simulink model "BACKUP"  (R2023b)
settings: Solver=VariableStepAuto  StartTime=0.0  StopTime=10.0  RelTol=1e-3
values from neighbouring files (symbols this model uses):
  C_PM = 1.758e-3    (= 0.001758)    [HVDCMMCInterconnectionParam.m]
  Carm = C_PM/Nb_PM    (= 4.88333333333e-05)    [HVDCMMCInterconnectionParam.m]
  Cfilter = 1/(Larm*wc2)    (= 4.78421193241e-05)    [HVDCMMCInterconnectionParam.m]
  Cg = 50e-9    (= 5e-08)    [HVDCMMCInterconnectionParam.m]
  Dd11 = Dd(1:nsw,1:nsw);        if(isempty(Dd11)) Dd11 = zeros(3,3); end    [DSS.m]    (also in DSS_test.m)
  Dd12 = Dd(1:nsw,nsw+1:end);    if(isempty(Dd12)) Dd12 = zeros(3,3); end    [DSS.m]    (also in DSS_test.m)
  Fnom = 50    [HVDCMMCInterconnectionParam.m]
  HRM = 2    [HVDCMMCInterconnectionParam.m]
  Ib_ac = (2/3)*Pnom/Vb_ac    [HVDCMMCInterconnectionParam.m]
  Ki_Ireg = 6    [HVDCMMCInterconnectionParam.m]
  Ki_Preg = 1.0    (= 1)    [HVDCMMCInterconnectionParam.m]
  Ki_Qreg = 1.0    (= 1)    [HVDCMMCInterconnectionParam.m]
  Ki_VDCreg = 100    [HVDCMMCInterconnectionParam.m]
  Kp_Ireg = 0.6    [HVDCMMCInterconnectionParam.m]
  Kp_Preg = 0.5/3    (= 0.166666666667)    [HVDCMMCInterconnectionParam.m]
  Kp_Qreg = 0.5/3    (= 0.166666666667)    [HVDCMMCInterconnectionParam.m]
  Kp_VDCreg = 4    [HVDCMMCInterconnectionParam.m]
  L_cable = 15e-3    (= 0.015)    [HVDCMMCInterconnectionParam.m]
  Larm = Larm_pu*(Zb_ac/(2*pi*Fnom))    [HVDCMMCInterconnectionParam.m]
  Lff = Larm_pu/2    (= 0.075)    [HVDCMMCInterconnectionParam.m]
  Limits_Ireg = [ 2.0  -2.0]    [HVDCMMCInterconnectionParam.m]
  Limits_Preg = [ 1.2, 0.8 ]    [HVDCMMCInterconnectionParam.m]
  Limits_Qreg = [ 0.25, -0.25 ]    [HVDCMMCInterconnectionParam.m]
  Limits_VDCreg = [ 2.0  -2.0]    [HVDCMMCInterconnectionParam.m]
  Lxfo = 0.12    [HVDCMMCInterconnectionParam.m]
  Nb_PM = 36    [HVDCMMCInterconnectionParam.m]
  Pnom = 1000e6    (= 1000000000)    [HVDCMMCInterconnectionParam.m]
  R_cable = 0.5    [HVDCMMCInterconnectionParam.m]
  R_startup = 400    [HVDCMMCInterconnectionParam.m]
  Rarm = Rarm_pu*Zb_ac    [HVDCMMCInterconnectionParam.m]
  Rff = Rarm_pu/2    (= 0.00075)    [HVDCMMCInterconnectionParam.m]
  Rfilter = 1/(Cfilter*w)*30    (= 1996.002)    [HVDCMMCInterconnectionParam.m]
  Rg = 100    [HVDCMMCInterconnectionParam.m]
  Rxfo = 0.003    [HVDCMMCInterconnectionParam.m]
  Ts = Ts_Control    (= 4e-05)    [HVDCMMCInterconnectionParam.m]
  Ts_Control = 40e-6    (= 4e-05)    [HVDCMMCInterconnectionParam.m]
  Ts_Power = 20e-6    (= 2e-05)    [HVDCMMCInterconnectionParam.m]
  Vb_ac = sqrt(2/3)*Vnom_sec    [HVDCMMCInterconnectionParam.m]
  Vc0_PM = 0    [HVDCMMCInterconnectionParam.m]
  Vnom_dc = 640e3    (= 640000)    [HVDCMMCInterconnectionParam.m]
  Vnom_prim = 400e3    (= 400000)    [HVDCMMCInterconnectionParam.m]
  Vnom_sec = 333e3    (= 333000)    [HVDCMMCInterconnectionParam.m]
  w = 2*pi*Fnom    (= 314.159265359)    [HVDCMMCInterconnectionParam.m]
  Zb_ac = Vb_ac/Ib_ac    [HVDCMMCInterconnectionParam.m]
undefined symbols (not defined in the file or in its folder): Ad1, Bd1, Cd1, DiscIntNeverNeededParam, gcbh, HrmOrd, Pcc, sps_AC, sps_ACDC, sps_rtmsupport, SYS, Ts_EMT
libraries: spsSeriesRLCBranchLib x22, simulink x20, spsCurrentMeasurementLib x13, spsControlledVoltageSourceLib x12, DQN_Lib x9, spsdq0toabcLib x3, powerlib_extras x3, spsGroundLib x3, spsBreakerLib x3, spsParallelRLCBranchLib x3, eeGeneralControl x2, dspspect3 x2
(part 2 of 5)

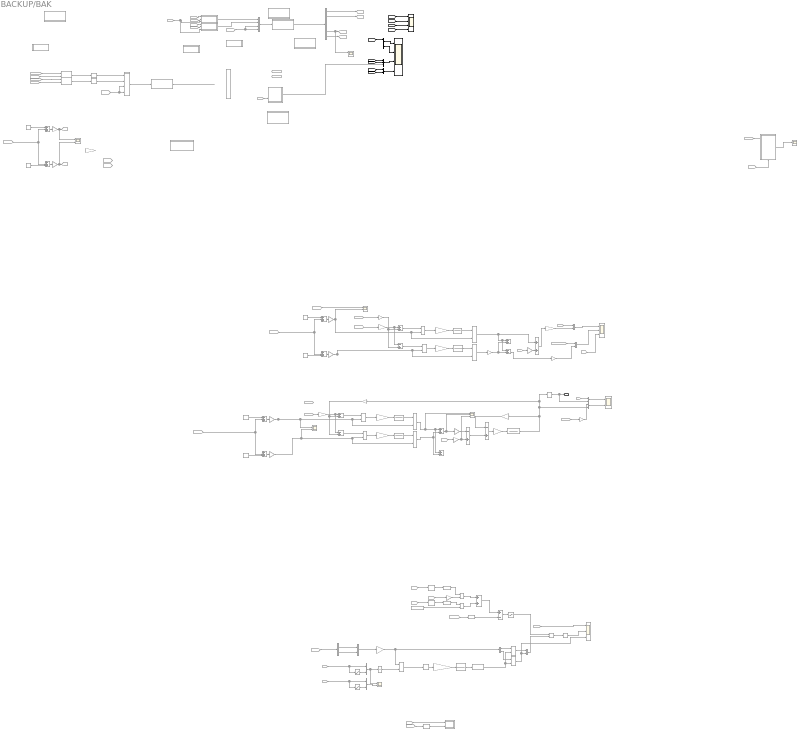
== system BACKUP/BAK ==
  3ph SM1 : Subsystem  Commented=on
  Add{,1,3,7,11} (5 alike) : Sum  Commented=on
  Add2 : Sum  Commented=on  Inputs=-+
  Add4 : Sum  Commented=on  Inputs=+-
  Add6 : Sum  Commented=on  Inputs=-+
  Add9 : Sum  Commented=on  Inputs=-+
  Compare To Constant1 : simulink/Logic and Bit Operations/Compare To Constant  Commented=on  relop=>  const=0.5  OutDataTypeStr=boolean
  Compare To Constant2 : simulink/Logic and Bit Operations/Compare To Constant  Commented=on  relop=<=  const=0.5  OutDataTypeStr=boolean
  Constant{1..4,74..75} (6 alike) : Constant  Commented=on
  Constant5 : Constant  Commented=on  Value=Vb_ac
  DQn->ABC1 : MATLAB Function  Commented=on  TreatAsAtomicUnit=on  SystemSampleTime=Ts_Power  mask{N=HRM}
      mask prompts: N "Harmonic order:"
  Data Type Conversion1 : DataTypeConversion  Commented=on  OutDataTypeStr=double  SaturateOnIntegerOverflow=off  RndMeth=Floor
  Data Type Conversion2 : DataTypeConversion  Commented=on  OutDataTypeStr=double  SaturateOnIntegerOverflow=off  RndMeth=Floor
  Delay : Delay  Commented=on  DelayLength=1  SampleTime=Ts_Power
  Delay1 : Delay  Commented=on  DelayLength=1  SampleTime=Ts_Power
  Delay3 : Subsystem  Commented=on
  Demux : Demux  Commented=on  Outputs=numel(sps_AC.outputs)/3
  Demux11 : Demux  Commented=on  Outputs=2
  Demux9 : Demux  Commented=on  Outputs=2
  Demux_DQNc_Mat : Subsystem  Commented=on  mask{nrOut=numel(sps_AC.outputs)/3}
      mask prompts: nrOut "Number of outputs [{C}]"
      mask init:
      | if(isempty(nrOut))
      |     Simulink.SubSystem.deleteContents(gcb);
      | else
      | 
      |     IndexOptionArray = cell(2,1);
      |     IndexOptionArray(1) = {'Select all'           };
      |     IndexOptionArray(2) = {'Index vector (dialog)'};
      | 
      |     PortHandles = get_param(gcb,'PortHandles');
      | 
      |     lenOut = length(PortHandles.Outport);
      | 
      |     if(nrOut ~= lenOut) % Important to avoid reinitialization of the block!
      | 
      |         Simulink.SubSystem.deleteContents(gcb);
      | 
      |         add_block('built-in/Inport',[gcb,strcat('/In',num2str(1))]);
      |         set_param([gcb,strcat('/In',num2str(1))],'position' , [50,65+1*50,90,85+1*50]);
      | 
      |         for i = 1 : nrOut
      |             add_block('simulink/Signal Routing/Selector',[gcb,strcat('/Sel',num2str(i))],...
      |                 'IndexOptionArray',IndexOptionArray,...
      |                 'NumberOfDimensions','2',...
      |                 'IndexOptions','Index vector (dialog),Select all',...
      |                 'Indices',strcat(num2str((i-1)*3+1),':',num2str((i-1)*3+3),', 1') ...
      |                 );
      |             set_param([gcb,strcat('/Sel',num2str(i))],'position' , [450,65+i*50,490,85+i*50])
      | 
      | 
      |             add_block('built-in/Outport',[gcb,strcat('/Out',num2str(i))]);
      |             set_param([gcb,strcat('/Out',num2str(i))],'position' , [750,65+i*50,790,85+i*50]);
      | 
      |             add_line(gcb,strcat('In',num2str(1),'/1'),  strcat('Sel',num2str(i),'/1'),'autorouting','on');
      |             add_line(gcb,strcat('Sel',num2str(i),'/1'), strcat('Out',num2str(i),'/1'),'autorouting','on');
      |         end
      | 
      |     end
      | 
      | end
      mask Display: disp(['{\color{red}\bf\fontsize{12}} [\{X_C\}]',newline,' DE-',newline,' MUX'], 'texmode','on');
  Discrete State-Space : Subsystem  Commented=on  mask{A=sps_AC.A, B=sps_AC.B, C=sps_AC.C, D=sps_AC.D, InitVec=sps_AC.x0, dt=Ts_Power}
      mask prompts: InitVec "Initial condition:"; dt "Time step (s):"
      mask init:
      | I = eye(size(A,1));
      | INVR = I/(I-A*dt/2);
      | Ad1 = INVR*(I+A*dt/2);
      | Bd1 = INVR*B*dt/2;
      | Cd1 = C*Ad1;
      | Dd11 = C*INVR*B*dt/2+D;
      | Dd12 = C*INVR*B*dt/2;
      settings: LibrarySourceBlock=|
      | spsSynchronousMachineModel/Discrete robust/State Space Model/Discretize
      | BE or Tustin
      mask Display: disp(['{\color{red}\bf\fontsize{12}x(t) = Ad*x(t-dt)+Bd*u(t)}',newline,'{\color{gray}\bf\fontsize{12}y(t) = Cd*x(t-dt)+Dd*u(t)}'], 'texmode','on');
  Discrete State-Space1 : Subsystem  Commented=on  mask{A=sps_AC.A, B=sps_AC.B, C=sps_AC.C, D=sps_AC.D, InitVec=sps_AC.x0, dt=Ts_Power}
      mask prompts: InitVec "Initial condition:"; dt "Time step (s):"
      mask init:
      | % I = eye(size(A,1));
      | % INVR = I/(I-A*dt/2);
      | % Ad1 = INVR*(I+A*dt/2);
      | % Bd1 = INVR*B*dt/2;
      | % Cd1 = C*Ad1;
      | % Cd = INVR*C*dt;
      | % Dd11 = C*INVR*B*dt/2+D;
      | % Dd12 = C*INVR*B*dt/2;
      settings: LibrarySourceBlock=|
      | spsSynchronousMachineModel/Discrete robust/State Space Model/Discretize
      | BE or Tustin
      mask Display: disp(['{\color{red}\bf\fontsize{12}x(t) = Ad*x(t-dt)+Bd*u(t)}',newline,'{\color{gray}\bf\fontsize{12}y(t) = Cd*x(t-dt)+Dd*u(t)}'], 'texmode','on');
  Discrete State-Space2 : Subsystem  Commented=on  mask{A=sps_AC.A, B=sps_AC.B, C=sps_AC.C, D=sps_AC.D, InitVec=[], dt=Ts, N=HRM, Ws=w}
      mask prompts: InitVec "Initial condition:"; dt "Time step (s):"; N "Order number:"; Ws "Angular frequency (rad/s);"
      mask init:
      | %Discretization of Continuous-Time Systems in the State Space with Numerical Integration Methods
      | 
      | method = 1;
      | 
      | % if(method)
      | % 
      | %     I = eye(size(A,1));
      | %     INVR = I/(I-A*dt/2);
      | %     Ad1 = INVR*(I+A*dt/2);
      | %     Bd1 = INVR*B*dt/2;
      | %     Cd1 = C*Ad1;
      | %     Dd1 = C*INVR*B*dt/2+D;
      | %     Dd12 = C*INVR*B*dt/2;
      | % 
      | % else
      | %     I = eye(size(A,1));
      | %     INVR = I/(I-A*dt/2);
      | %     Ad1 = INVR*(I+A*dt/2);
      | %     Bd1 = INVR*B;
      | %     Cd1 = C*INVR*dt;
      | %     Dd1 = Cd1*B/2;
      | % end
      | 
      |     if(method)
      | 
      |         I = eye(size(A,1));
      |         INVR = I/(I-A*dt/2);
      |         Ad1 = INVR*(I+A*dt/2);
      |         Bd1 = INVR*B;
      |         Cd1 = C*INVR*dt;
      |         Dd1 = Cd1*B/2;
      |     else
      |         Ad1 = A;
      |         Bd1 = B;
      |         Cd1 = C;
      |         Dd1 = D;
      |     end
      | 
      | %Calculating the PNZ matrices
      | 
      |     a = -0.5+0.866i;
      |     a2 = -0.5-0.866i;
      |     Sas = [1,a,a2;1,a2,a;1,1,1]/3;
      | 
      |     arows = size(Ad1,1)/3; %signal size
      |     acols = size(Ad1,2)/3; %signal size
      | 
      |     brows = size(Bd1,1)/3; %signal size
      |     bcols = size(Bd1,2)/3; %signal size
      | 
      |     crows = size(Cd1,1)/3; %signal size
      |     ccols = size(Cd1,2)/3; %signal size
      | 
      |     d1rows = size(Dd1,1)/3; %signal size
      |     d1cols = size(Dd1,2)/3; %signal size
      | 
      |     %%%%%%%%%%%%%%%%%%%%%%% Check for inconsistencies  %%%%%%%%%%%%%%%%%%%%%%%
      | 
      |     szMatA = size(A,1);
      |     iL = eye(szMatA);
      |     szMatiL = size(iL,1);
      | 
      |     if(szMatiL ~= szMatA || size(A,1) ~= size(A,2) || size(iL,1) ~= size(iL,2))
      |         error('[Int_DQN_Mat/swFeedback] check matrix A size!');
      |     end
      | 
      |     if(arows ~= brows || acols ~= ccols || crows ~= d1rows || bcols ~= d1cols)
      |         error('[Int_DQN_Mat/Initialize] the sizes of the state-space matrices!');
      |     end
      | 
      |     %%%%%%%%%%%%%%%%%%%%%%%%%%%%%%%%%%%%%%%%%%%%%%%%%%%%%%%%%%%%%%%
      | 
      | 
      |     %%%%%%%%%%%%%%%%%%%%%%% A --> Bpnz %%%%%%%%%%%%%%%%%%%%%%%
      |     Adc = complex(zeros(3*arows,3*acols));
      | 
      |     for i = 1 : arows
      |         for j = 1 : acols
      |             Adc((1:3) + (i-1)*3,(1:3) + (j-1)*3) = Sas*Ad1((1:3) + (i-1)*3,(1:3) + (j-1)*3)/Sas;
      |             %Adc((1:3) + (i-1)*3,(1:3) + (j-1)*3) = diag(diag(real(Adc((1:3) + (i-1)*3,(1:3) + (j-1)*3))));
      |             %Adc((1:3) + (i-1)*3,(1:3) + (j-1)*3) = diag(diag((Adc((1:3) + (i-1)*3,(1:3) + (j-1)*3))));
      | 
      |         end
      |     end
      |     %%%%%%%%%%%%%%%%%%%%%%%%%%%%%%%%%%%%%%%%%%%%%%%%%%%%%%%%%%%%%%%
      | 
      |     %%%%%%%%%%%%%%%%%%%%%%% B --> Bpnz %%%%%%%%%%%%%%%%%%%%%%%
      | 
      |     Bdc = complex(zeros(3*brows,3*bcols));
      | 
      |     for i = 1 : brows
      |         for j = 1 : bcols
      |             Bdc((1:3) + (i-1)*3,(1:3) + (j-1)*3) = Sas*Bd1((1:3) + (i-1)*3,(1:3) + (j-1)*3)/Sas;
      |             %Bdc((1:3) + (i-1)*3,(1:3) + (j-1)*3) = diag(diag(real(Bdc((1:3) + (i-1)*3,(1:3) + (j-1)*3))));
      |             %Bdc((1:3) + (i-1)*3,(1:3) + (j-1)*3) = diag(diag((Bdc((1:3) + (i-1)*3,(1:3) + (j-1)*3))));
      | 
      |         end
      |     end
      |     %%%%%%%%%%%%%%%%%%%%%%%%%%%%%%%%%%%%%%%%%%%%%%%%%%%%%%%%%%%%%%%
      | 
      |     %%%%%%%%%%%%%%%%%%%%%%% C --> Cpnz %%%%%%%%%%%%%%%%%%%%%%%
      | 
      |     Cdc = complex(zeros(3*crows,3*ccols));
      | 
      |     for i = 1 : crows
      |         for j = 1 : ccols
      |             Cdc((1:3) + (i-1)*3,(1:3) + (j-1)*3) = Sas*Cd1((1:3) + (i-1)*3,(1:3) + (j-1)*3)/Sas;
      |             %Cdc((1:3) + (i-1)*3,(1:3) + (j-1)*3) = diag(diag(real(Cdc((1:3) + (i-1)*3,(1:3) + (j-1)*3))));
      |             %Cdc((1:3) + (i-1)*3,(1:3) + (j-1)*3) = diag(diag((Cdc((1:3) + (i-1)*3,(1:3) + (j-1)*3))));
      |         end
      |     end
      |     %%%%%%%%%%%%%%%%%%%%%%%%%%%%%%%%%%%%%%%%%%%%%%%%%%%%%%%%%%%%%%%
      | 
      |     
      |     %%%%%%%%%%%%%%%%%%%%%%% D1 --> Cpnz %%%%%%%%%%%%%%%%%%%%%%%
      | 
      |     Ddc = complex(zeros(3*d1rows,3*d1cols));
      | 
      |     for i = 1 : d1rows
      |         for j = 1 : d1cols
      |             Ddc((1:3) + (i-1)*3,(1:3) + (j-1)*3) = Sas*Dd1((1:3) + (i-1)*3,(1:3) + (j-1)*3)/Sas;
      |             %Ddc1((1:3) + (i-1)*3,(1:3) + (j-1)*3) = diag(diag(real(Ddc1((1:3) + (i-1)*3,(1:3) + (j-1)*3))));
      |             %Ddc((1:3) + (i-1)*3,(1:3) + (j-1)*3) = diag(diag((Ddc((1:3) + (i-1)*3,(1:3) + (j-1)*3))));
      |         end
      |     end
      |     %%%%%%%%%%%%%%%%%%%%%%%%%%%%%%%%%%%%%%%%%%%%%%%%%%%%%%%%%%%%%%%
      | 
      |     Adc(abs(Adc)<2*eps) = 0;
      |     Bdc(abs(Bdc)<2*eps) = 0;
      |     Cdc(abs(Cdc)<2*eps) = 0;
      |     Ddc(abs(Ddc)<2*eps) = 0;
      | 
      |     % I = eye(size(Adc,1));
      |     % INVR = I/(I-Adc*dt/2);
      |     % Adc = INVR*(I+Adc*dt/2);
      |     % Bdc = INVR*Bdc;
      |     % Cdc = Cdc*INVR*dt;
      |     % Ddc = Cdc*Bdc/2;
      | 
      |     if(method ~= 1)
      |         I = eye(size(Adc,1));
      |         INVR = I/(I-Adc*dt/2);
      |         Adc = INVR*(I+Adc*dt/2);
      |         Bdc = INVR*Bdc;
      |         Cdc = Cdc*INVR*dt;
      |         Ddc = Cdc*Bdc/2;
      |     end
      | 
      | 
      | 
      | 
      |     InitVec_c = complex(zeros(brows*3,N+1));
      | 
      | 
      |     if(~isempty(InitVec))
      |         if(mod(numel(InitVec),3)~=0) error('[SS_DQNc_Mat] InitVec with wrong size --> needs to be a multiple of 3!'); end
      | 
      |         for k = 1 : numel(InitVec)/3
      |             InitVec_c((k-1)*3+1:(k-1)*3+3,1) = Sas*InitVec((k-1)*3+1:(k-1)*3+3)*exp(+1i*Ws*dt);
      |         end
      |     end
      settings: LibrarySourceBlock=|
      | spsSynchronousMachineModel/Discrete robust/State Space Model/Discretize
      | BE or Tustin
      mask Display: disp(['{\color{red}\bf\fontsize{12}x(t) = Ad*x(t-dt)+Bd*u(t)}',newline,'{\color{gray}\bf\fontsize{12}y(t) = Cd*x(t-dt)+Dd*u(t)}'], 'texmode','on');
  Discrete State-Space4 : Subsystem  Commented=on  mask{A=sps_AC.A, B=sps_AC.B, C=sps_AC.C, D=sps_AC.D, InitVec=sps_AC.x0, dt=Ts_Power, DQSYM=on, N=HRM, Ws=w}
      mask prompts: InitVec "Initial condition:"; dt "Time step (s):"; N "Harmonic number:"; Ws "Angular frequency (1/rad):"
      mask init: same as BACKUP/Discrete State-Space2
      settings: LibrarySourceBlock=|
      | spsSynchronousMachineModel/Discrete robust/State Space Model/Discretize
      | BE or Tustin
      mask Display: disp(['{\color{red}\bf\fontsize{12}x(t) = Ad*x(t-dt)+Bd*u(t)}',newline,'{\color{gray}\bf\fontsize{12}y(t) = Cd*x(t-dt)+Dd*u(t)}'], 'texmode','on');
  Discrete State-Space5 : Subsystem  Commented=on  SystemSampleTime=Ts_Power  mask{A=sps_AC.A, B=sps_AC.B, C=sps_AC.C, D=sps_AC.D, InitVec=sps_AC.x0, dt=Ts_Power, DQSYM=off, N=HRM, Ws=w}
      mask prompts: InitVec "Initial condition:"; dt "Time step (s):"; N "Harmonic number:"; Ws "Angular frequency (1/rad):"
      mask init: same as BACKUP/Discrete State-Space2
      settings: MinAlgLoopOccurrences=on
      settings: LibrarySourceBlock=|
      | spsSynchronousMachineModel/Discrete robust/State Space Model/Discretize
      | BE or Tustin
      mask Callback DQSYM:
      | EMT = get_param(gcb,'DQSYM');
      | 
      | if(strcmp(EMT,'on'))
      |    set_param(gcb,'MaskVisibilities',{'on','on','on','on','on','on','on','on','on'});
      | else
      |    set_param(gcb,'MaskVisibilities',{'on','on','on','on','on','on','on','off','off'});
      | end
      mask Display: disp(['{\color{red}\bf\fontsize{12}x(t) = Ad*x(t-dt)+Bd*u(t)}',newline,'{\color{gray}\bf\fontsize{12}y(t) = Cd*x(t-dt)+Dd*u(t)}'], 'texmode','on');
  Discrete-Time Integrator : DiscreteIntegrator  Commented=on  IntegratorMethod=Integration: Trapezoidal  SampleTime=Ts_Power  ICPrevOutput=DiscIntNeverNeededParam  ICPrevScaledInput=DiscIntNeverNeededParam
  Discrete-Time Integrator1 : DiscreteIntegrator  Commented=on  IntegratorMethod=Integration: Trapezoidal  SampleTime=Ts_Power  ICPrevOutput=DiscIntNeverNeededParam  ICPrevScaledInput=DiscIntNeverNeededParam
  Discrete-Time Integrator2 : DiscreteIntegrator  Commented=on  IntegratorMethod=Integration: Trapezoidal  SampleTime=Ts_EMT  ICPrevOutput=DiscIntNeverNeededParam  ICPrevScaledInput=DiscIntNeverNeededParam
  Discrete-Time Integrator3 : DiscreteIntegrator  Commented=on  IntegratorMethod=Integration: Trapezoidal  SampleTime=Ts_EMT  ICPrevOutput=DiscIntNeverNeededParam  ICPrevScaledInput=DiscIntNeverNeededParam
  Discrete-Time Integrator4 : DiscreteIntegrator  Commented=on  IntegratorMethod=Integration: Trapezoidal  SampleTime=Ts_EMT  ICPrevOutput=DiscIntNeverNeededParam  ICPrevScaledInput=DiscIntNeverNeededParam
  Discrete-Time Integrator5 : DiscreteIntegrator  Commented=on  IntegratorMethod=Integration: Trapezoidal  gainval=1  SampleTime=Ts_Power  UpperSaturationLimit=5000  LowerSaturationLimit=500  ICPrevOutput=DiscIntNeverNeededParam  ICPrevScaledInput=DiscIntNeverNeededParam
  From1 : From  Commented=on  GotoTag=Uref_ABC  TagVisibility=global
  From100 : From  Commented=on  GotoTag=Uref_ABC  TagVisibility=global
  From101 : From  Commented=on  GotoTag=Id_abc  TagVisibility=global
  From102 : From  Commented=on  GotoTag=Isec  TagVisibility=global
  From103 : From  Commented=on  GotoTag=Id_abc  TagVisibility=global
  From104 : From  Commented=on  GotoTag=Vp_ss
  From105 : From  Commented=on  GotoTag=Vsec_ss
  From106 : From  Commented=on  GotoTag=Uref_ABC  TagVisibility=global
  From108 : From  Commented=on  GotoTag=Id_abc  TagVisibility=global
  From{80,109..110,112} (4 alike) : From  Commented=on  GotoTag=Vdc1  TagVisibility=global
  From111 : From  Commented=on  GotoTag=Ig_abc  TagVisibility=global
  From14 : From  Commented=on  GotoTag=Vsec_ABC
  From16 : From  Commented=on  GotoTag=wt0  TagVisibility=global
  From18 : From  Commented=on  GotoTag=Blk  TagVisibility=global
  From24 : From  Commented=on  GotoTag=VSRC_C
  From25 : From  Commented=on  GotoTag=U_Brk1_C
  From26 : From  Commented=on  GotoTag=wt0  TagVisibility=global
  From27 : From  Commented=on  GotoTag=U_Brk1_C
  From28 : From  Commented=on  GotoTag=Brk1_On  TagVisibility=global
  From29 : From  Commented=on  GotoTag=U_Brk2_C
  From30 : From  Commented=on  GotoTag=Brk2_On  TagVisibility=global
  From33 : From  Commented=on  GotoTag=m1_dq  TagVisibility=global
  From34 : From  Commented=on  GotoTag=Vsec  TagVisibility=global
  From35 : From  Commented=on  GotoTag=U_Brk1_C
  From37 : From  Commented=on  GotoTag=Brk1_On  TagVisibility=global
  From39 : From  Commented=on  GotoTag=U_Brk1
  From49 : From  Commented=on  GotoTag=Brk2_On  TagVisibility=global
  From51 : From  Commented=on  GotoTag=U_Brk2
  From54 : From  Commented=on  GotoTag=Uref_ABC
  From75 : From  Commented=on  GotoTag=Blk  TagVisibility=global
  From76 : From  Commented=on  GotoTag=V12_Ap  TagVisibility=global
  From77 : From  Commented=on  GotoTag=Vsec  TagVisibility=global
  From78 : From  Commented=on  GotoTag=Uref_Ap  TagVisibility=global
  From79 : From  Commented=on  GotoTag=I_Ap  TagVisibility=global
  From82 : From  Commented=on  GotoTag=Blk  TagVisibility=global
  From83 : From  Commented=on  GotoTag=I_Bp  TagVisibility=global
  From84 : From  Commented=on  GotoTag=Uref_p  TagVisibility=global
  From97 : From  Commented=on  GotoTag=Idc1  TagVisibility=global
  Gain{7,10..12} (4 alike) : Gain  Commented=on
  Gain{2,4,8,13} (4 alike) : Gain  Commented=on  Gain=0.5
  Gain14 : Gain  Commented=on  Gain=Nb_PM
  Gain15 : Gain  Commented=on  Gain=1/(C_PM*Nb_PM)
  Gain{3,17..18,21} (4 alike) : Gain  Commented=on  Gain=1/(Carm)
  Gain27 : Gain  Commented=on  Gain=1/(Larm)
  Gain28 : Gain  Commented=on  Gain=Rarm
  Gain6 : Gain  Commented=on  Gain=1/0.001
  Gain9 : Gain  Commented=on  Gain=1/3
  Goto1 : Goto  Commented=on  GotoTag=U_Brk1
  Goto2 : Goto  Commented=on  GotoTag=U_Brk2
  Goto27 : Goto  Commented=on  GotoTag=mp  TagVisibility=global
  Goto28 : Goto  Commented=on  GotoTag=mn  TagVisibility=global
  Goto3 : Goto  Commented=on  GotoTag=Iprim_SS
  Goto4 : Goto  Commented=on  GotoTag=Isec_SS
  Goto5 : Goto  Commented=on  GotoTag=U_Brk1_C
  Goto6 : Goto  Commented=on  GotoTag=U_Brk2_C
  I->pu{1..6,22,28} (8 alike) : Gain  Commented=on  Gain=1/2  SaturateOnIntegerOverflow=on  OutDataTypeStr=Inherit: Same as input  ParamDataTypeStr=Inherit: Same as input
  I->pu12 : Gain  Commented=on  Gain=0.5  SaturateOnIntegerOverflow=on  OutDataTypeStr=Inherit: Same as input  ParamDataTypeStr=Inherit: Same as input
  MATLAB Function : MATLAB Function  Commented=on  TreatAsAtomicUnit=on  SystemSampleTime=Ts_Power
      settings: MinAlgLoopOccurrences=on
  MATLAB Function1 : MATLAB Function  Commented=on  TreatAsAtomicUnit=on  SystemSampleTime=Ts_Power
      settings: MinAlgLoopOccurrences=on
  MMC_ABC : Subsystem  Commented=on
      settings: PortSchema="{\"entries\":[{\"content\":{\"sides\":[{\"content\":{\"connectorIds\":[\"In1\",\"In2\",\"Out3\",\"Out4\"]},\"type\":\"ConnectorPlacement.EquallySpacedRectSide\",\"uuid\":\"684906a0-21fb-41a6-b3c5-f77045d253ac\"},{\"content\":{\"connectorIds\":[\"Out1\"],\"side\":\"RIGHT\"},\"type\":\"ConnectorPlacement.EquallySpacedRectSide\",\"uuid\":\"9d85a733-ae48-4655-9ff6-63838a16e886\"},{\"content\":{\"connectorIds\":[\"In3\",\"Out2\"],\"side\":\"TOP\"},\"type\":\"ConnectorPlacement.EquallySpacedRectSide\",\"uuid\":\"d076c62e-607a-4519-bbe3-5591fb02f9d6\"},{\"content\":{\"connectorIds\":[\"In4\"],\"side\":\"BOTTOM\"},\"type\":\"ConnectorPlacement.EquallySpacedRectSide\",\"uuid\":\"e22e3e72-7b47-4480-8e5d-6e636dd9340b\"}]},\"type\":\"ConnectorPlacement.EquallySpacedConnector\",\"uuid\":\"6c134aa3-44e6-4e9e-9485-00d5bee37874\"}],\"packageUris\":[\"http://schema.mathworks.com/mf0/Connector/R2020b\"],\"version\":\"1.0\"}"
  Min5 : MinMax  Commented=on  Inputs=2
  Mux : Mux  Commented=on  Inputs=numel(sps_AC.inputs)/3
  Mux1 : Mux  Inputs=2
  Mux{18,22..24,32..33,35..36} (8 alike) : Mux  Commented=on  Inputs=2
  Mux2 : Mux  Inputs=2
  Mux3 : Mux  Inputs=3
  Mux4 : Mux  Inputs=2
  Mux_DQNc_Mat : Subsystem  Commented=on  mask{nrInp=4}
      mask prompts: nrInp "Number of inputs [{C}]"
      mask init:
      | %blocks = find_system(gcb,'LookUnderMasks','on','FollowLinks','on')
      | %set_param(gcb, 'MaskSelfModifiable', 'on');
      | 
      | % if(SSM == [])
      | %     Simulink.SubSystem.deleteContents(gcb);
      | % else
      | 
      | if(isempty(nrInp))
      |     Simulink.SubSystem.deleteContents(gcb);
      | else
      | 
      |     nrOut = 1;
      | 
      | 
      | PortHandles = get_param(gcb,'PortHandles');
      | lenInp = length(PortHandles.Inport);
      | lenOut = length(PortHandles.Inport);
      | 
      | if(nrInp ~= lenInp)
      |     %disp('ENTERED')
      |     Simulink.SubSystem.deleteContents(gcb);
      | %     add_block('simulink/Continuous/State-Space', [gcb,'/ss_block'], 'A','SS.A', 'B','SS.B', 'C','SS.C', 'D','SS.D', 'X0','X0')
      | %     set_param([gcb,'/ss_block'],'position' , [350,100,450,150])
      | 
      | 
      | 
      |         add_block('simulink/Math Operations/Matrix Concatenate',[gcb,'/Mux'], 'NumInputs',num2str(nrInp), 'ConcatenateDimension',num2str(1));
      |         set_param([gcb,'/Mux'],'position' , [200,100,250,100+nrInp*50])
      |         
      | %         add_block('built-in/Demux',[gcb,'/Demux'], 'Outputs',num2str(nrOut));
      | %         set_param([gcb,'/Demux'],'position' , [500,100,550,100+nrOut*50])
      | 
      | 
      |         for i = 1 : nrInp
      |             add_block('built-in/Inport',[gcb,strcat('/In',num2str(i))]);
      |             set_param([gcb,strcat('/In',num2str(i))],'position' , [50,65+i*50,90,85+i*50]);
      |             add_line(gcb,strcat('In',num2str(i),'/1'),strcat('Mux/',num2str(i)),'autorouting','on');
      |         end
      | 
      |         for i = 1 : nrOut
      |             add_block('built-in/Outport',[gcb,strcat('/Out',num2str(i))]);
      |             set_param([gcb,strcat('/Out',num2str(i))],'position' , [750,65+i*50,790,85+i*50]);
      |             add_line(gcb,strcat('Mux/',num2str(i)), strcat('Out',num2str(i),'/1'),'autorouting','on');
      |         end
      | 
      | 
      | %     add_line(gcb, 'Mux/1', 'ss_block/1')
      | %     add_line(gcb, 'ss_block/1', 'Demux/1')
      | 
      | end
      | 
      | end
      mask Display: disp(['{\color{red}\bf\fontsize{12}} [\{X_C\}]',newline,' MUX'], 'texmode','on');
  Product{1..13} (13 alike) : Product  Commented=on
  SS_DQNc_Mat_Dicrete : Subsystem  Commented=on  AncestorBlock=DQN_Lib/SS_DQNc_Mat_Dicrete  mask{A=sps_AC.A, B=sps_AC.B, C=sps_AC.C, D=sps_AC.D, InitVec=sps_AC.x0, dt=Ts, N=HRM, Ws=w}
      mask prompts: InitVec "Initial condition:"; dt "Time step (s):"; N "Harmonic order:"; Ws "Angular frequency (rad/s):"
      mask init:
      | I = eye(size(A,1));
      |     
      |     INVR = I/(I-A*dt/2);
      |     
      |     Ad = INVR*(I+A*dt/2);
      |     
      |     Bd = INVR*B;
      |     
      |     Cd = C*INVR*dt;
      |     
      |     Dd = Cd*B/2;
      | 
      |     % dt2 = dt/2;
      |     % 
      |     % a = -0.5+0.866i;
      |     % a2 = -0.5-0.866i;
      |     % Sas = [1,a,a2;1,a2,a;1,1,1]/3;
      |     % 
      |     % arows = size(Ad,1)/3; %signal size
      |     % acols = size(Ad,2)/3; %signal size
      |     % 
      |     % brows = size(Bd,1)/3; %signal size
      |     % bcols = size(Bd,2)/3; %signal size
      |     % 
      |     % crows = size(Cd,1)/3; %signal size
      |     % ccols = size(Cd,2)/3; %signal size
      |     % 
      |     % drows = size(Dd,1)/3; %signal size
      |     % dcols = size(Dd,2)/3; %signal size
      |     % 
      |     % %%%%%%%%%%%%%%%%%%%%%%% Check for inconsistencies  %%%%%%%%%%%%%%%%%%%%%%%
      |     % 
      |     % szMatA = size(A,1);
      |     % iL = eye(szMatA);
      |     % szMatiL = size(iL,1);
      |     % 
      |     % if(szMatiL ~= szMatA || size(A,1) ~= size(A,2) || size(iL,1) ~= size(iL,2))
      |     %     error('[Int_DQN_Mat/swFeedback] check matrix A size!');
      |     % end
      |     % 
      |     % if(arows ~= brows || acols ~= ccols || crows ~= drows || bcols ~= dcols)
      |     %     error('[Int_DQN_Mat/Initialize] the sizes of the state-space matrices!');
      |     % end
      |     % 
      |     % %%%%%%%%%%%%%%%%%%%%%%%%%%%%%%%%%%%%%%%%%%%%%%%%%%%%%%%%%%%%%%%
      |     % 
      |     % %%%%%%%%%%%%%%%%%%%%%%% A --> Bpnz %%%%%%%%%%%%%%%%%%%%%%%
      |     % Adc = complex(zeros(3*arows,3*acols));
      |     % 
      |     % for i = 1 : arows
      |     %     for j = 1 : acols
      |     %         Adc((1:3) + (i-1)*3,(1:3) + (j-1)*3) = Sas*Ad((1:3) + (i-1)*3,(1:3) + (j-1)*3)/Sas;
      |     %         %Adc((1:3) + (i-1)*3,(1:3) + (j-1)*3) = diag(diag(real(Adc((1:3) + (i-1)*3,(1:3) + (j-1)*3))));
      |     %     end
      |     % end
      |     % %%%%%%%%%%%%%%%%%%%%%%%%%%%%%%%%%%%%%%%%%%%%%%%%%%%%%%%%%%%%%%%
      |     % 
      |     % %%%%%%%%%%%%%%%%%%%%%%% B --> Bpnz %%%%%%%%%%%%%%%%%%%%%%%
      |     % 
      |     % Bdc = complex(zeros(3*brows,3*bcols));
      |     % 
      |     % for i = 1 : brows
      |     %     for j = 1 : bcols
      |     %         Bdc((1:3) + (i-1)*3,(1:3) + (j-1)*3) = Sas*Bd((1:3) + (i-1)*3,(1:3) + (j-1)*3)/Sas;
      |     %         %Bdc((1:3) + (i-1)*3,(1:3) + (j-1)*3) = diag(diag(real(Bdc((1:3) + (i-1)*3,(1:3) + (j-1)*3))));
      |     %     end
      |     % end
      |     % %%%%%%%%%%%%%%%%%%%%%%%%%%%%%%%%%%%%%%%%%%%%%%%%%%%%%%%%%%%%%%%
      |     % 
      |     % %%%%%%%%%%%%%%%%%%%%%%% C --> Cpnz %%%%%%%%%%%%%%%%%%%%%%%
      |     % 
      |     % Cdc = complex(zeros(3*crows,3*ccols));
      |     % 
      |     % for i = 1 : crows
      |     %     for j = 1 : ccols
      |     %         Cdc((1:3) + (i-1)*3,(1:3) + (j-1)*3) = Sas*Cd((1:3) + (i-1)*3,(1:3) + (j-1)*3)/Sas;
      |     %         %Cdc((1:3) + (i-1)*3,(1:3) + (j-1)*3) = diag(diag(real(Cdc((1:3) + (i-1)*3,(1:3) + (j-1)*3))));
      |     %     end
      |     % end
      |     % %%%%%%%%%%%%%%%%%%%%%%%%%%%%%%%%%%%%%%%%%%%%%%%%%%%%%%%%%%%%%%%
      |     % 
      |     % %%%%%%%%%%%%%%%%%%%%%%% C --> Cpnz %%%%%%%%%%%%%%%%%%%%%%%
      |     % 
      |     % Ddc = complex(zeros(3*drows,3*dcols));
      |     % 
      |     % for i = 1 : drows
      |     %     for j = 1 : dcols
      |     %         Ddc((1:3) + (i-1)*3,(1:3) + (j-1)*3) = Sas*Dd((1:3) + (i-1)*3,(1:3) + (j-1)*3)/Sas;
      |     %         %Ddc((1:3) + (i-1)*3,(1:3) + (j-1)*3) = diag(diag(real(Ddc((1:3) + (i-1)*3,(1:3) + (j-1)*3))));
      |     %     end
      |     % end
      |     % %%%%%%%%%%%%%%%%%%%%%%%%%%%%%%%%%%%%%%%%%%%%%%%%%%%%%%%%%%%%%%%
      |     % 
      |     % 
      |     % 
      |     % Adc(abs(Adc)<2*eps) = 0;
      |     % Bdc(abs(Bdc)<2*eps) = 0;
      |     % Cdc(abs(Cdc)<2*eps) = 0;
      |     % Ddc(abs(Ddc)<2*eps) = 0;
      |     % 
      |     % % Adc = real(Adc);
      |     % % Bdc = real(Bdc);
      |     % % Cdc = real(Cdc);
      |     % % Ddc = real(Ddc);
      |     % 
      |     % 
      |     % InitVec_c = complex(zeros(brows*3,N+1));
      |     % 
      |     % 
      |     % if(~isempty(InitVec))
      |     %     if(mod(numel(InitVec),3)~=0) error('[SS_DQNc_Mat] InitVec with wrong size --> needs to be a multiple of 3!'); end
      |     % 
      |     %     for k = 1 : numel(InitVec)/3
      |     %         InitVec_c((k-1)*3+1:(k-1)*3+3,1) = Sas*InitVec((k-1)*3+1:(k-1)*3+3);
      |     %     end
      |     % end
      |     % 
      |     % 
      |     % 
      |     %
      settings: LibrarySourceBlock=|
      | spsSynchronousMachineModel/Discrete robust/State Space Model/Discretize
      | BE or Tustin
      mask Display: disp(['{\color{red}\bf\fontsize{12}x(t) = Ad*x(t-dt)+Bd*u(t)}',newline,'{\color{gray}\bf\fontsize{12}y(t) = Cd*x(t-dt)+Dd*u(t)}'], 'texmode','on');
  SW1 : Subsystem  Commented=on
  Saturation : Saturate  Commented=on  UpperLimit=inf  LowerLimit=0
  Saturation1 : Saturate  Commented=on  UpperLimit=inf  LowerLimit=0
  Saturation3 : Saturate  Commented=on  UpperLimit=inf  LowerLimit=0
  Scope{,2,4..5,7,10} (6 alike) : Scope  Commented=on  NumInputPorts=2
  Scope1 : Scope  Commented=on
  Scope12 : Scope  Commented=on  NumInputPorts=3
  Scope3 : Scope  Commented=on  NumInputPorts=3
  Scope6 : Scope  NumInputPorts=4
  Scope8 : Scope  Commented=on  NumInputPorts=3
  Scope9 : Scope  NumInputPorts=4
  Selector1 : Selector  Commented=on  InputPortWidth=3  IndexOptions=Index vector (dialog)  Indices=[1]  OutputSizes=1
  Selector5 : Selector  Commented=on  InputPortWidth=3  IndexOptions=Index vector (dialog)  Indices=1  OutputSizes=1
  Subsystem1 : Subsystem  Commented=on  TreatAsAtomicUnit=on  SystemSampleTime=Ts_Power
      settings: MinAlgLoopOccurrences=on
  Subsystem2 : Subsystem  Commented=on  TreatAsAtomicUnit=on  SystemSampleTime=Ts_Power
      settings: MinAlgLoopOccurrences=on
  Subsystem3 : Subsystem  Commented=on  TreatAsAtomicUnit=on  SystemSampleTime=Ts_Power
  Subsystem4 : Subsystem  Commented=on  TreatAsAtomicUnit=on  SystemSampleTime=Ts_Power
      settings: MinAlgLoopOccurrences=on
  Subsystem8 : Subsystem  Commented=on  TreatAsAtomicUnit=on  SystemSampleTime=Ts_Power
      settings: MinAlgLoopOccurrences=on
  Subtract1 : Sum  Commented=on  Inputs=+-+
  Subtract2 : Sum  Commented=on  Inputs=+-+
  Subtract3 : Sum  Commented=on  Inputs=+-+
  Subtract4 : Sum  Commented=on  Inputs=+++
  Subtract5 : Sum  Commented=on  Inputs=+++
  Subtract6 : Sum  Commented=on  Inputs=+++
  Subtract7 : Sum  Commented=on  Inputs=+-
  Sum of Elements : Sum  Commented=on  Inputs=+
  Sum of Elements1 : Sum  Commented=on  Inputs=+
  Sum1 : Sum  Commented=on  InputSameDT=on  SaturateOnIntegerOverflow=on  OutDataTypeStr=Inherit: Same as first input
  Sum3 : Sum  Commented=on  Inputs=-+  InputSameDT=on  SaturateOnIntegerOverflow=on  OutDataTypeStr=Inherit: Same as first input
  Sum4 : Sum  Commented=on  Inputs=-+  InputSameDT=on  SaturateOnIntegerOverflow=on  OutDataTypeStr=Inherit: Same as first input
  Sum8 : Sum  Commented=on  Inputs=1  InputSameDT=on  SaturateOnIntegerOverflow=on  OutDataTypeStr=Inherit: Same as first input
  Unit Delay4 : UnitDelay  Commented=on  SampleTime=Ts_Power  HasFrameUpgradeWarning=on
  Idc : Outport
  wires:
  From51/1 -> Subsystem1/1(Ubrk)
  From49/1 -> Subsystem1/2(com)
  Discrete State-Space5/1(Y) -> Demux/1
  From16/1 -> Subsystem1/3(Ubrk1), Subsystem2/3(Ubrk1)  "theta"
  Subsystem2/1(Vcalc) -> Mux/1
  ? -> DQn->ABC1/1(Xdcpnz_c)  "[N+1,18 (6+6+6)]"
  ? -> Goto5/1
  Discrete State-Space4/1(Y) -> ?
  ? -> Goto6/1
  Delay/1 -> Mux_DQNc_Mat/1(In1)
  Delay1/1 -> Mux_DQNc_Mat/2(In2)
  From24/1 -> Mux_DQNc_Mat/3(In3), Mux_DQNc_Mat/4(In4)
  MATLAB Function1/1(y) -> Delay1/1
  MATLAB Function/1(y) -> Delay/1
  Mux1/1 -> Scope6/2
  From30/1 -> MATLAB Function1/2(com)
  Demux/6 -> Goto4/1
  From35/1 -> MATLAB Function/1(u)
  From29/1 -> MATLAB Function1/1(u)
  Demux/2 -> Goto2/1
  From26/1 -> DQn->ABC1/2(tho)  "theta"
  DQn->ABC1/1(Xabc) -> Mux3/3  "Iprim_DQN"
  From37/1 -> Subsystem2/2(com)
  Subsystem1/1(Vcalc) -> Mux/2
  Demux/1 -> Goto1/1
  Mux_DQNc_Mat/1(Out1) -> Discrete State-Space4/1(U)
  From28/1 -> MATLAB Function/2(com)
  From14/1 -> Mux/3, Mux/4
  Mux/1 -> Discrete State-Space5/1(U)
  [Iprim_SS] -> Mux3/2
  [Iprim] -> Scope9/4  "Iprim"
  Mux4/1 -> Scope6/1
  Mux2/1 -> Scope6/4
  From54/1 -> Subtract2/2, Subtract5/2
  [Vprim] -> Scope9/2  "Vprim"
  [Vsec] -> Scope9/1  "Vsec"
  [Isec] -> Mux2/1
  Mux3/1 -> Scope6/3
  [Iprim] -> Mux3/1
  Demux/5 -> Scope7/1, Goto3/1
  From34/1 -> MMC_ABC/4(Vsec)
  Constant74/1 -> Subtract2/1
  From39/1 -> Subsystem2/1(Ubrk)
  [U_Brk1] -> Mux4/1
  Subtract2/1 -> I->pu22/1
  I->pu22/1 -> Scope2/1, Goto27/1
  [Isec_SS] -> Mux2/2
  I->pu28/1 -> Scope2/2, Goto28/1
  Subtract5/1 -> I->pu28/1
  Constant75/1 -> Subtract5/3
  From33/1 -> MMC_ABC/1(m_dq1)
  MMC_ABC/1(Vconv) -> Scope1/1
  [Isec] -> Scope9/3  "Isec"
  Gain11/1 -> Mux36/1
  I->pu2/1 -> Scope12/3, Sum3/2
  Gain17/1 -> Discrete-Time Integrator2/1  "dVp_M"
  Mux35/1 -> Scope10/1
  Gain18/1 -> Discrete-Time Integrator3/1  "dVn_M"
  From84/1 -> Scope4/1
  From112/1 -> Scope3/3
  From100/1 -> Subtract6/2, Subtract1/2
  Product10/1 -> Gain17/1
  Subtract4/1 -> I->pu5/1
  From106/1 -> Subtract4/2, Subtract3/2
  Product3/1 -> Add2/1, Add1/1, Sum1/1  "Iabc_B22 (A)"
  Gain28/1 -> Sum4/1
  Add6/1 -> Product7/1
  Discrete-Time Integrator1/1 -> Product8/1  "Vn_M"
  Gain9/1 -> Mux32/2
  Product8/1 -> Gain7/1
  Discrete-Time Integrator/1 -> Product3/1  "Vp_M"
  I->pu12/1 -> Sum1/2
  Subtract1/1 -> I->pu1/1
  Gain2/1 -> Add6/1, Add3/1
  Constant4/1 -> Subtract4/3
  Add11/1 -> Scope12/2, I->pu6/1  "dVp_M"
  Gain7/1 -> Add2/2, Add1/2
  Sum3/1 -> Sum4/2
  Gain12/1 -> Add9/2, Add7/2
  Discrete-Time Integrator4/1 -> Mux36/2, Sum of Elements1/1, Gain12/1, Gain28/1  "dVp_M"
  Gain13/1 -> Add9/1, Add7/1
  From97/1 -> Mux35/1  "Idc_EMT"
  Product13/1 -> Add11/2, Add4/2
  Add2/1 -> Gain8/1
  I->pu5/1 -> Scope5/2, Product12/2, Product13/2
  Constant3/1 -> Subtract6/3
  From104/1 -> Mux32/1
  Sum4/1 -> Gain27/1
  From102/1 -> Gain2/1  "Igd"
  Product7/1 -> Gain21/1
  Gain27/1 -> Discrete-Time Integrator4/1
  From105/1 -> Mux33/1
  Subtract3/1 -> I->pu4/1
  From108/1 -> Gain11/1  "diff_EMT"
  Add3/1 -> Product4/1  "prod"
  I->pu3/1 -> Product8/2, Product7/2
  From110/1 -> I->pu2/1
  Gain21/1 -> Discrete-Time Integrator1/1  "dVn_M"
  Mux36/1 -> Scope10/2
  Sum1/1 -> Gain9/1
  Add9/1 -> Product12/1
  Constant2/1 -> Subtract3/1
  From111/1 -> Gain13/1
  I->pu6/1 -> Sum3/1
  Subtract6/1 -> I->pu3/1
  Product12/1 -> Gain18/1
  Sum of Elements1/1 -> Mux35/2, Idc/1
  From101/1 -> Gain10/1
  Mux32/1 -> Scope3/1
  ? -> Subtract6/1, Subtract1/3
  Gain3/1 -> Discrete-Time Integrator/1  "dVp_M"
  From109/1 -> I->pu12/1
  Gain8/1 -> Mux33/2
  Product11/1 -> Scope12/1, Add4/1, Add11/1  "Iabc_B22 (A)"
  I->pu4/1 -> Scope5/1, Product11/2, Product10/2
  Gain10/1 -> Add6/2, Add3/2
  Constant1/1 -> Subtract1/1
  I->pu1/1 -> Product3/2, Product4/2, Scope4/2
  Mux33/1 -> Scope3/2
  Discrete-Time Integrator3/1 -> Product13/1  "Vn_M"
  Add7/1 -> Product10/1  "prod"
  Discrete-Time Integrator2/1 -> Product11/1  "Vp_M"
  Product4/1 -> Gain3/1
  Selector1/1 -> SW1/2(Uref_1ph)
  From1/1 -> Selector1/1
  Sum of Elements/1 -> Scope8/2
  From75/1 -> Compare To Constant1/1
  From77/1 -> Selector5/1
  Compare To Constant2/1 -> Data Type Conversion1/1
  Data Type Conversion1/1 -> Product2/1
  Gain4/1 -> Product5/2
  Data Type Conversion2/1 -> Product5/1
  Add/1 -> Subtract7/1
  From80/1 -> Gain4/1
  Product5/1 -> Add/1
  Product1/1 -> Sum8/1
  From82/1 -> Compare To Constant2/1
  Mux22/1 -> Scope/1, Unit Delay4/1
  From78/1 -> Demux11/1
  Demux11/1 -> Mux24/1  "Uref"
  Constant5/1 -> Product2/2
  Saturation3/1 -> Mux22/2
  From79/1 -> Saturation3/1, Mux22/1
  From18/1 -> SW1/1(Blk)
  Demux9/2 -> Product9/1
  Subtract7/1 -> Saturation/1
  Mux18/1 -> Scope/2
  Demux11/2 -> Mux24/2  "Ublk"
  Saturation1/1 -> Mux18/2
  Product9/1 -> Scope8/3, Mux23/2  "Vbl"
  Demux9/1 -> Product6/1
  Sum8/1 -> Gain15/1
  Delay3/1(Vc) -> Product9/2, Product6/2
  Gain14/1 -> Demux9/1, Product1/1
  Product2/1 -> Add/2
  Unit Delay4/1 -> Product1/2
  Min5/1 -> Sum of Elements/1
  Mux24/1 -> Gain14/1
  Gain15/1 -> Discrete-Time Integrator5/1
  Compare To Constant1/1 -> Data Type Conversion2/1
  Product6/1 -> Mux23/1  "Vin"
  Mux23/1 -> Min5/2
  Selector5/1 -> Subtract7/2
  From76/1 -> Scope8/1  "Target"
  Discrete-Time Integrator5/1 -> Delay3/1(In1)
  Saturation/1 -> Min5/1
  From83/1 -> Saturation1/1, Mux18/1

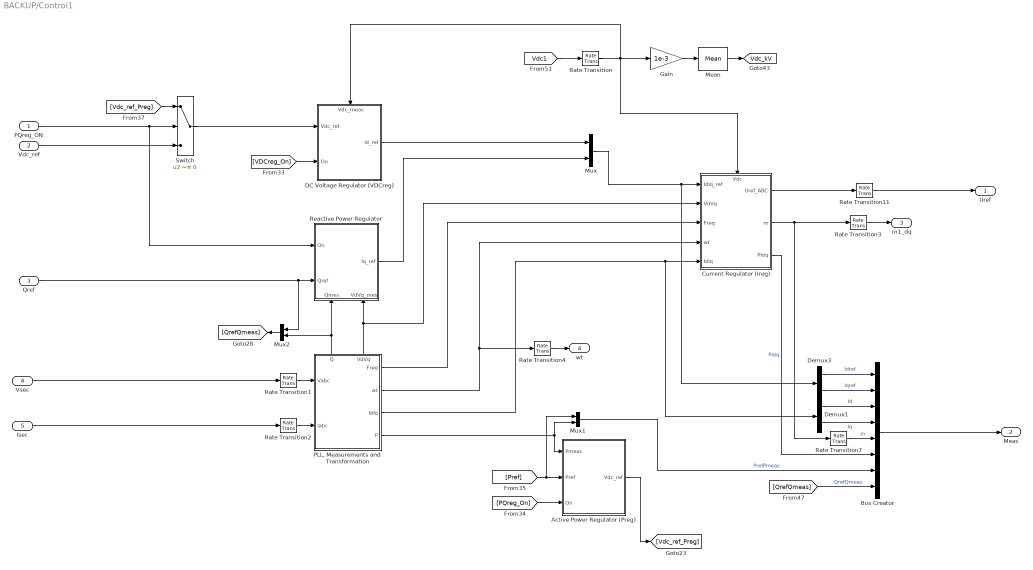
== system BACKUP/Control1 ==
  PQreg_ON : Inport
  Vdc_ref : Inport  Port=2
  Qref : Inport  Port=3
  Vsec : Inport  Port=4
  Isec : Inport  Port=5
  Active Power Regulator (Preg) : Subsystem
  Bus Creator : BusCreator  Inputs=8
  Current Regulator (Ireg) : Subsystem
      settings: PortSchema="{\"entries\":[{\"content\":{\"sides\":[{\"content\":{\"connectorIds\":[\"In1\",\"In2\",\"In3\",\"In4\",\"In5\"]},\"type\":\"ConnectorPlacement.EquallySpacedRectSide\",\"uuid\":\"46fff04e-1450-479d-b460-437d90e99f23\"},{\"content\":{\"connectorIds\":[\"Out1\",\"Out2\",\"Out3\"],\"side\":\"RIGHT\"},\"type\":\"ConnectorPlacement.EquallySpacedRectSide\",\"uuid\":\"1fecc714-62d0-4152-98c9-212d930a5fef\"},{\"content\":{\"connectorIds\":[\"In6\"],\"side\":\"TOP\"},\"type\":\"ConnectorPlacement.EquallySpacedRectSide\",\"uuid\":\"861e6320-ec6e-4c2a-8449-e621a478dd1e\"}]},\"type\":\"ConnectorPlacement.EquallySpacedConnector\",\"uuid\":\"2e901dc7-e129-44fe-b6c0-1fa97996cfbd\"}],\"packageUris\":[\"http://schema.mathworks.com/mf0/Connector/R2020b\"],\"version\":\"1.0\"}"
  DC Voltage Regulator (VDCreg) : Subsystem
      settings: PortSchema="{\"entries\":[{\"content\":{\"sides\":[{\"content\":{\"connectorIds\":[\"In1\",\"In2\"]},\"type\":\"ConnectorPlacement.EquallySpacedRectSide\",\"uuid\":\"c20f24de-2933-46ae-a608-0dc6cbdc22c5\"},{\"content\":{\"connectorIds\":[\"Out1\"],\"side\":\"RIGHT\"},\"type\":\"ConnectorPlacement.EquallySpacedRectSide\",\"uuid\":\"78958689-3494-4241-b4e6-c71b7d261298\"},{\"content\":{\"connectorIds\":[\"In3\"],\"side\":\"TOP\"},\"type\":\"ConnectorPlacement.EquallySpacedRectSide\",\"uuid\":\"05cc66e2-c7d6-407f-b011-a28bc71811d6\"}]},\"type\":\"ConnectorPlacement.EquallySpacedConnector\",\"uuid\":\"0d848e7c-ac8e-4664-bac3-455723337427\"}],\"packageUris\":[\"http://schema.mathworks.com/mf0/Connector/R2020b\"],\"version\":\"1.0\"}"
  Demux1 : Demux  Outputs=2
  Demux3 : Demux  Outputs=2
  Gain : Gain  Gain=1e-3
  Mean : spsMeanLib/Mean  Freq=Fnom/3  Vinit=0  Ts=Ts_Control
  Mux : Mux  Inputs=2
  Mux1 : Mux  Inputs=2
  Mux2 : Mux  Inputs=2
  "PLL, Measurements and Transformation" : Subsystem
      settings: PortSchema="{\"entries\":[{\"content\":{\"sides\":[{\"content\":{\"connectorIds\":[\"In1\",\"In2\"]},\"type\":\"ConnectorPlacement.EquallySpacedRectSide\",\"uuid\":\"b10cca13-b0c2-430a-b17c-db71eb4f1a3c\"},{\"content\":{\"connectorIds\":[\"Out1\",\"Out2\",\"Out3\",\"Out4\"],\"side\":\"RIGHT\"},\"type\":\"ConnectorPlacement.EquallySpacedRectSide\",\"uuid\":\"355382eb-bc30-4f3c-94e5-48c8b9c2ecfd\"},{\"content\":{\"connectorIds\":[\"Out5\",\"Out6\"],\"side\":\"TOP\"},\"type\":\"ConnectorPlacement.EquallySpacedRectSide\",\"uuid\":\"77f94122-ff4d-41eb-b55d-9b38525f3ab4\"}]},\"type\":\"ConnectorPlacement.EquallySpacedConnector\",\"uuid\":\"46538cda-22c7-46a2-9cc9-63f6dc7214f2\"}],\"packageUris\":[\"http://schema.mathworks.com/mf0/Connector/R2020b\"],\"version\":\"1.0\"}"
  Rate Transition{,1..2,7} (4 alike) : RateTransition  OutPortSampleTime=Ts_Control
  Rate Transition11 : RateTransition  OutPortSampleTime=Ts_Power
  Rate Transition3 : RateTransition  OutPortSampleTime=Ts_Power
  Rate Transition4 : RateTransition  OutPortSampleTime=Ts_Power
  Reactive Power Regulator : Subsystem
      settings: PortSchema="{\"entries\":[{\"content\":{\"sides\":[{\"content\":{\"connectorIds\":[\"In1\",\"In2\"]},\"type\":\"ConnectorPlacement.EquallySpacedRectSide\",\"uuid\":\"eeeb811d-908b-486e-b0fa-0b5fd0d6695a\"},{\"content\":{\"connectorIds\":[\"Out1\"],\"side\":\"RIGHT\"},\"type\":\"ConnectorPlacement.EquallySpacedRectSide\",\"uuid\":\"28c9bf02-c5ab-433a-87a9-c17e67d0c029\"},{\"content\":{\"side\":\"TOP\"},\"type\":\"ConnectorPlacement.EquallySpacedRectSide\",\"uuid\":\"fdca837a-4079-4910-a6d7-edbb284eaa51\"},{\"content\":{\"connectorIds\":[\"In3\",\"In4\"],\"side\":\"BOTTOM\"},\"type\":\"ConnectorPlacement.EquallySpacedRectSide\",\"uuid\":\"d2fa5805-110b-4a78-bf6e-301fd334a724\"}]},\"type\":\"ConnectorPlacement.EquallySpacedConnector\",\"uuid\":\"cbc8ea8f-55f5-4ff6-b34f-d5812b415dcf\"}],\"packageUris\":[\"http://schema.mathworks.com/mf0/Connector/R2020b\"],\"version\":\"1.0\"}"
  Switch : Switch  Criteria=u2 ~= 0  SaturateOnIntegerOverflow=off  InputSameDT=off
  Uref : Outport
  Meas : Outport  Port=2
  m1_dq : Outport  Port=3
  wt : Outport  Port=4
  tag scope: Vdc_kV=global
  wires:
  Mux1/1 -> Bus Creator/7  "PrefPmeas"
  "PLL, Measurements and Transformation"/4(P) -> Mux1/2, Active Power Regulator (Preg)/1(Pmeas)
  DC Voltage Regulator (VDCreg)/1(Id_ref) -> Mux/1
  "PLL, Measurements and Transformation"/2(wt) -> Rate Transition4/1, Current Regulator (Ireg)/4(wt)
  Demux1/1 -> Bus Creator/3  "Id"
  Vsec/1 -> Rate Transition1/1
  "PLL, Measurements and Transformation"/6(VdVq) -> Reactive Power Regulator/4(VdVq_mes), Current Regulator (Ireg)/2(VdVq)
  Mux2/1 -> [QrefQmeas]
  Rate Transition11/1 -> Uref/1
  "PLL, Measurements and Transformation"/5(Q) -> Mux2/2, Reactive Power Regulator/3(Qmes)
  [Pref] -> Active Power Regulator (Preg)/2(Pref), Mux1/1
  Isec/1 -> Rate Transition2/1
  [PQreg_On] -> Active Power Regulator (Preg)/3(On)
  [QrefQmeas] -> Bus Creator/8  "QrefQmeas"
  Current Regulator (Ireg)/2(m) -> Rate Transition3/1, Rate Transition7/1
  Demux3/2 -> Bus Creator/2  "Iqref"
  Rate Transition7/1 -> Bus Creator/5  "m"
  [Vdc_ref_Preg] -> Switch/1
  Demux3/1 -> Bus Creator/1  "Idref"
  Mux/1 -> Demux3/1, Current Regulator (Ireg)/1(IdIq_ref)
  Switch/1 -> DC Voltage Regulator (VDCreg)/1(Vdc_ref)
  Current Regulator (Ireg)/3(PIdq) -> Bus Creator/6  "PIdq"
  [Vdc1] -> Rate Transition/1
  PQreg_ON/1 -> Reactive Power Regulator/1(On), Switch/2
  Rate Transition1/1 -> "PLL, Measurements and Transformation"/1(Vabc)
  "PLL, Measurements and Transformation"/1(Freq) -> Current Regulator (Ireg)/3(Freq)
  Vdc_ref/1 -> Switch/3
  Active Power Regulator (Preg)/1(Vdc_ref) -> [Vdc_ref_Preg]
  Gain/1 -> Mean/1
  Mean/1 -> [Vdc_kV]
  Rate Transition2/1 -> "PLL, Measurements and Transformation"/2(Iabc)
  Rate Transition/1 -> DC Voltage Regulator (VDCreg)/3(Vdc_meas), Current Regulator (Ireg)/6(Vdc), Gain/1
  [VDCreg_On] -> DC Voltage Regulator (VDCreg)/2(On)
  Demux1/2 -> Bus Creator/4  "Iq"
  "PLL, Measurements and Transformation"/3(IdIq) -> Current Regulator (Ireg)/5(IdIq), Demux1/1
  Qref/1 -> Mux2/1, Reactive Power Regulator/2(Qref)
  Current Regulator (Ireg)/1(Uref_ABC) -> Rate Transition11/1
  Bus Creator/1 -> Meas/1
  Reactive Power Regulator/1(Iq_ref) -> Mux/2
  Rate Transition3/1 -> m1_dq/1
  Rate Transition4/1 -> wt/1

== system BACKUP/DC & converter 3 ==
  Add : Sum
  Cinv : spsSeriesRLCBranchLib/Series RLC Branch  LConnTagsString=__new0  RConnTagsString=__new0  BranchType=RC  Resistance=1e-3  Inductance=1e-3  SetiL0=off  InitialCurrent=0  Capacitance=C_PM/Nb_PM*3  Setx0=off  InitialVoltage=Vnom_dc/2  Measurements=None
  Cinv1 : spsSeriesRLCBranchLib/Series RLC Branch  LConnTagsString=__new0  RConnTagsString=__new0  BranchType=RC  Resistance=1e-3  Inductance=1e-3  SetiL0=off  InitialCurrent=0  Capacitance=C_PM/Nb_PM*3  Setx0=off  InitialVoltage=Vnom_dc/2  Measurements=None
  CnDC : spsSeriesRLCBranchLib/Series RLC Branch  LConnTagsString=__new0  RConnTagsString=__new0  BranchType=RC  Resistance=Rg  Inductance=1e-3  SetiL0=off  InitialCurrent=0  Capacitance=Cg  Setx0=off  InitialVoltage=Vnom_dc/2  Measurements=None
  CpDC : spsSeriesRLCBranchLib/Series RLC Branch  LConnTagsString=__new0  RConnTagsString=__new0  BranchType=RC  Resistance=Rg  Inductance=1e-3  SetiL0=off  InitialCurrent=0  Capacitance=Cg  Setx0=off  InitialVoltage=Vnom_dc/2  Measurements=None
  Current Measurement1 : spsCurrentMeasurementLib/Current Measurement  PhasorSimulation=off  OutputType=Complex  PSBequivalent=0
  Current Measurement2 : spsCurrentMeasurementLib/Current Measurement  PhasorSimulation=off  OutputType=Complex  PSBequivalent=0
  Gain : Gain  Gain=0.5
  Gain1 : Gain  Gain=-1
  Ground2 : spsGroundLib/Ground  LConnTagsString=a
  Ground4 : spsGroundLib/Ground  LConnTagsString=a
  Voltage Measurement2 : spsVoltageMeasurementLib/Voltage Measurement  PhasorSimulation=off  OutputType=Complex  PSBequivalent=0
  Zcable1_1 : spsSeriesRLCBranchLib/Series RLC Branch  LConnTagsString=__new0  RConnTagsString=__new0  BranchType=RL  Resistance=R_cable/2  Inductance=L_cable/2  SetiL0=off  InitialCurrent=0  Capacitance=1e-6  Setx0=off  InitialVoltage=0  Measurements=None
  Zcable1_2 : spsSeriesRLCBranchLib/Series RLC Branch  LConnTagsString=__new0  RConnTagsString=__new0  BranchType=RL  Resistance=R_cable/2  Inductance=L_cable/2  SetiL0=off  InitialCurrent=0  Capacitance=1e-6  Setx0=off  InitialVoltage=0  Measurements=None
  Zcable2_1 : spsSeriesRLCBranchLib/Series RLC Branch  LConnTagsString=__new0  RConnTagsString=__new0  BranchType=RL  Resistance=R_cable/2  Inductance=L_cable/2  SetiL0=off  InitialCurrent=0  Capacitance=1e-6  Setx0=off  InitialVoltage=0  Measurements=None
  Zcable2_2 : spsSeriesRLCBranchLib/Series RLC Branch  LConnTagsString=__new0  RConnTagsString=__new0  BranchType=RL  Resistance=R_cable/2  Inductance=L_cable/2  SetiL0=off  InitialCurrent=0  Capacitance=1e-6  Setx0=off  InitialVoltage=0  Measurements=None
  Zcable5 : spsSeriesRLCBranchLib/Series RLC Branch  LConnTagsString=__new0  RConnTagsString=__new0  BranchType=RL  Resistance=1e-2+1e-3  Inductance=1e-4  SetiL0=off  InitialCurrent=0  Capacitance=1e-6  Setx0=off  InitialVoltage=0  Measurements=None
  Zcable6 : spsSeriesRLCBranchLib/Series RLC Branch  LConnTagsString=__new0  RConnTagsString=__new0  BranchType=RL  Resistance=1e-2+1e-3  Inductance=1e-4  SetiL0=off  InitialCurrent=0  Capacitance=1e-6  Setx0=off  InitialVoltage=0  Measurements=None
  1 : PMIOPort  Side=Left
  2 : PMIOPort  Port=2  Side=Left
  3 : PMIOPort  Port=3  Side=Right
  4 : PMIOPort  Port=4  Side=Right
  tag scope: Idc1=global, Vdc1=global
  wires:
  Voltage Measurement2/1 -> [Vdc1]
  Current Measurement2/1 -> Add/1
  Current Measurement1/1 -> Gain1/1
  Add/1 -> Gain/1
  Gain/1 -> [Idc1]
  Gain1/1 -> Add/2
  connections:
  Cinv/RConn1 -- Cinv1/LConn1 -- Ground2/LConn1
  CpDC/RConn1 -- Ground4/LConn1 -- CnDC/LConn1
  Zcable2_1/RConn1 -- CnDC/RConn1 -- Current Measurement1/RConn1 -- Voltage Measurement2/LConn2
  Zcable2_2/RConn1 -- Zcable2_1/LConn1
  Zcable1_1/RConn1 -- Voltage Measurement2/LConn1 -- Current Measurement2/RConn1 -- CpDC/LConn1
  1/RConn1 -- Current Measurement2/LConn1
  Zcable1_1/LConn1 -- Zcable1_2/RConn1
  Cinv1/RConn1 -- Zcable2_2/LConn1 -- Zcable6/RConn1
  Zcable1_2/LConn1 -- Cinv/LConn1 -- Zcable5/LConn1
  Current Measurement1/LConn1 -- 2/RConn1
  3/RConn1 -- Zcable5/RConn1
  4/RConn1 -- Zcable6/LConn1
